simulink model "test_plant_B_2013B"  (R2013b)
settings: Solver=ode45  StartTime=0.0  StopTime=sim_run  FixedStep=0.001  RelTol=1e-3
undefined symbols (not defined in the file): Standard_Devices, UDP_Protocol, zh_step
libraries: rtwinlib x1, dspnetwork x1
settings Model: CovModelRefEnable=off  Creator=Anony  LastModifiedBy=Anony
settings DataIOCC: SaveFormat=StructureWithTime
settings DebuggingCC: UnderspecifiedInitializationDetection=Simplified  MergeDetectMultiDrivingBlocksExec=error  SolverPrmCheckMsg=none  FrameProcessingCompatibilityMsg=error
settings HardwareCC: ProdBitPerPointer=64  ProdLargestAtomicFloat=Float  ProdIntDivRoundTo=Zero  ProdEndianess=LittleEndian  ProdHWDeviceType=Specified
settings GRTTargetCC: CodeReplacementLibrary=C89/C90 (ANSI)  GeneratePreprocessorConditionals=Use local settings

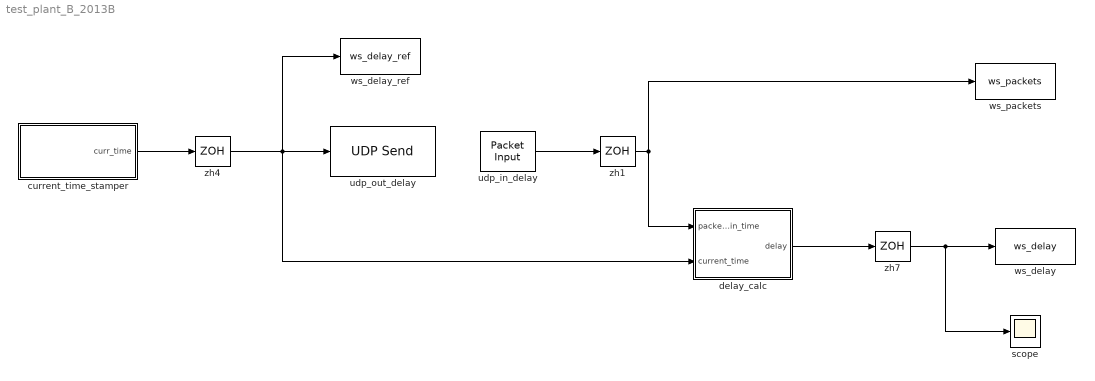
== system test_plant_B_2013B ==
  current_time_stamper : MATLAB Function  TreatAsAtomicUnit=on
      settings: PermitHierarchicalResolution=ParametersOnly
  delay_calc : Subsystem
  scope : Scope
      settings: TimeRange=auto  MaxDataPoints=5000  SaveToWorkspace=off  SaveName=ScopeData  YMin=-5009.625  YMax=45036.625  SampleTime=-1
  udp_in_delay : rtwinlib/Packet Input  SampleTime=0.001  MaxMissedTicks=inf  ShowMissedTicks=off  YieldWhenWaiting=off  DrvName=Standard_Devices/UDP_Protocol  DrvAddress=27000  DrvOptions=[2468394756 27000]  PacketSize=8  DataTypes='double'  ShowReady=off  ShowError=off  PacketID=1  ByteOrder=1  ShowTimestamp=off
      settings: AttributesFormatString=Standard Devices\nUDP Protocol [6978h]
  udp_out_delay : dspnetwork/UDP Send  remoteURL='147.32.183.4'  remotePort=28000  localURL='0.0.0.0'  localPortSource=Automatically determine  localPort=27000  sampletime=-1  separateLengthPort=0
  ws_delay : ToWorkspace  VariableName=ws_delay  SaveFormat=Timeseries  SampleTime=-1
  ws_delay_ref : ToWorkspace  VariableName=ws_delay_ref  SaveFormat=Timeseries  SampleTime=-1
  ws_packets : ToWorkspace  VariableName=ws_packets  SaveFormat=Timeseries  SampleTime=-1
  zh1 : ZeroOrderHold  SampleTime=zh_step
  zh4 : ZeroOrderHold  SampleTime=zh_step
  zh7 : ZeroOrderHold  SampleTime=zh_step
  wires:
  zh4/1 -> udp_out_delay/1, delay_calc/2(current_time), ws_delay_ref/1
  current_time_stamper/1(curr_time) -> zh4/1
  udp_in_delay/1 -> zh1/1
  zh1/1 -> delay_calc/1(packet_in_time), ws_packets/1
  zh7/1 -> scope/1, ws_delay/1
  delay_calc/1(delay) -> zh7/1

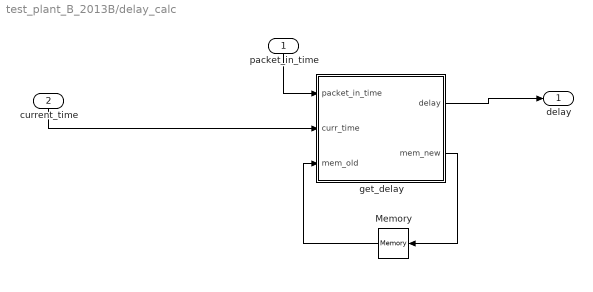
== system test_plant_B_2013B/delay_calc ==
  packet_in_time : Inport
  current_time : Inport  Port=2
  Memory : Memory
  get_delay : MATLAB Function  TreatAsAtomicUnit=on
      settings: PermitHierarchicalResolution=ParametersOnly
  delay : Outport
  wires:
  get_delay/2(mem_new) -> Memory/1
  get_delay/1(delay) -> delay/1
  Memory/1 -> get_delay/3(mem_old)
  current_time/1 -> get_delay/2(curr_time)
  packet_in_time/1 -> get_delay/1(packet_in_time)

== matlab function test_plant_B_2013B/current_time_stamper ==
  data: curr_time output
function curr_time = fcn()
%#codegen

coder.extrinsic('get_current_time'); 

     
% pause(0.01);
curr_time = 0;
curr_time = get_current_time();

== matlab function test_plant_B_2013B/delay_calc/get_delay ==
  data: delay output; packet_in_time input; curr_time input; mem_old input; mem_new output
function [delay,mem_new] = fcn(packet_in_time,...
                               curr_time,...
                               mem_old)
%#codegen

mem_new = 0;

if(packet_in_time > 0)
    mem_new = packet_in_time;
    if(mem_old ~= packet_in_time)
        delay = curr_time - packet_in_time;
    else
        delay = 0; % losst packet 
    end
else
    delay = -5; % no input received
    
end
